simulink model "dcm5"  (R2023a)
settings: Solver=ode45  StartTime=0.0  StopTime=2  RelTol=1e-3  EnableMultiTasking=on
InitFcn:
  | [dcm, cont] = dcm5_init
undefined symbols (not defined in the file or in its folder): cont, dcm
settings Model: Creator=jkempkes  LastModifiedBy=herranz
settings SolverCC: AlgebraicLoopSolver=TrustRegion
settings DataIOCC: LimitDataPoints=on  SaveFormat=Array  SignalLoggingSaveFormat=ModelDataLogs  ReturnWorkspaceOutputs=off  SignalLoggingName=sigsOut
settings OptimizationCC: BooleanDataType=off  LifeSpan=inf
settings DebuggingCC: SaveWithParameterizedLinksMsg=none  UnderspecifiedInitializationDetection=Classic  MergeDetectMultiDrivingBlocksExec=none  SignalResolutionControl=TryResolveAllWithWarning  MultiTaskDSMMsg=warning  MultiTaskCondExecSysMsg=none  UnconnectedInputMsg=warning  UnconnectedOutputMsg=warning  UnconnectedLineMsg=warning  SFUnexpectedBacktrackingDiag=warning  SFNoUnconditionalDefaultTransitionDiag=warning  SFExecutionAtInitializationDiag=none  ArithmeticOperatorsInVariantConditions=warning
settings HardwareCC: ProdBitPerPointer=32  ProdBitPerSizeT=32  ProdBitPerPtrDiffT=32  ProdLargestAtomicFloat=None  ProdIntDivRoundTo=Undefined  ProdEndianess=Unspecified  ProdWordSize=32  ProdHWDeviceType=32-bit Generic  TargetUnknown=on
settings ModelReferenceCC: PropagateSignalLabelsOutOfModel=off
settings SFSimCC: SimUseLocalCustomCode=off  CustomCodeUndefinedFunction=UseInterfaceOnly
settings RTWCC: RTWUseLocalCustomCode=off
settings CodeAppCC: StateflowObjectComments=on
settings GRTTargetCC: TargetLangStandard=C89/C90 (ANSI)  CombineOutputUpdateFcns=off  GRTInterface=on
settings ConfigComp: CovMetricSettings=dw  CovSaveCumulativeToWorkspaceVar=on  CovSaveSingleToWorkspaceVar=on  CovExternalEMLEnable=off

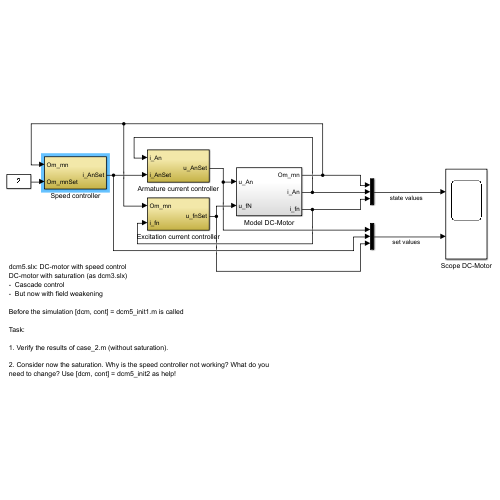
[thumbnail: Simulink's stored preview of the top-level diagram]
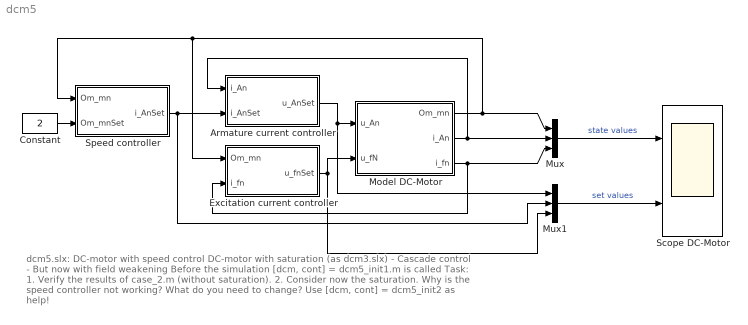
== system dcm5 ==
  note: dcm5.slx: DC-motor with speed control
      | DC-motor with saturation (as dcm3.slx)
      | -  Cascade control
      | -  But now with field weakening
      |
      | Before the simulation [dcm, cont] = dcm5_init1.m is called
      |
      | Task:
      |
      | 1. Verify the results of case_2.m (without saturation).
      |
      | 2. Consider now the saturation. Why is the speed controller not working? What do you need to change? Use [dcm, cont] = dcm5_init2 as help!
  Armature current controller : Subsystem
  Constant : Constant  Value=2
  Excitation current controller : Subsystem
  Model DC-Motor : Subsystem
  Mux : Mux  Inputs=3
  Mux1 : Mux  Inputs=3
  Scope DC-Motor : Scope  NumInputPorts=2
  Speed controller : Subsystem
  wires:
  Mux/1 -> Scope DC-Motor/1  "state values"
  Model DC-Motor/1(Om_mn) -> Mux/1, Speed controller/1(Om_mn), Excitation current controller/1(Om_mn)
  Model DC-Motor/2(i_An) -> Mux/2, Armature current controller/1(i_An)
  Model DC-Motor/3(i_fn) -> Mux/3, Excitation current controller/2(i_fn)
  Speed controller/1(i_AnSet) -> Armature current controller/2(i_AnSet), Mux1/2
  Armature current controller/1(u_AnSet) -> Model DC-Motor/1(u_An), Mux1/1
  Constant/1 -> Speed controller/2(Om_mnSet)
  Excitation current controller/1(u_fnSet) -> Model DC-Motor/2(u_fN), Mux1/3
  Mux1/1 -> Scope DC-Motor/2  "set values"

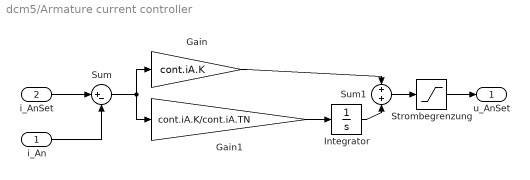
== system dcm5/Armature current controller ==
  i_An : Inport
  i_AnSet : Inport  Port=2
  Gain : Gain  Gain=cont.iA.K  SaturateOnIntegerOverflow=on  OutDataTypeStr=Inherit: Same as input  ParamDataTypeStr=Inherit: Same as input
  Gain1 : Gain  Gain=cont.iA.K/cont.iA.TN  SaturateOnIntegerOverflow=on  OutDataTypeStr=Inherit: Same as input  ParamDataTypeStr=Inherit: Same as input
  Integrator : Integrator  LimitOutput=on  UpperSaturationLimit=cont.u_Anmax  LowerSaturationLimit=-cont.u_Anmax
  Strombegrenzung : Saturate  UpperLimit=cont.u_Anmax  LowerLimit=-cont.u_Anmax
  Sum : Sum  Inputs=|+-  InputSameDT=on  SaturateOnIntegerOverflow=on  OutDataTypeStr=Inherit: Same as first input
  Sum1 : Sum  InputSameDT=on  SaturateOnIntegerOverflow=on  OutDataTypeStr=Inherit: Same as first input
  u_AnSet : Outport  InitialOutput=0
  wires:
  Strombegrenzung/1 -> u_AnSet/1
  i_An/1 -> Sum/2
  Sum/1 -> Gain1/1, Gain/1
  i_AnSet/1 -> Sum/1
  Sum1/1 -> Strombegrenzung/1
  Gain/1 -> Sum1/1
  Integrator/1 -> Sum1/2
  Gain1/1 -> Integrator/1

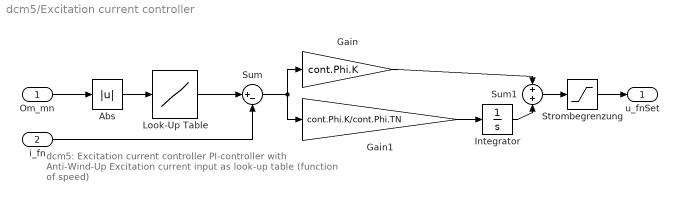
== system dcm5/Excitation current controller ==
  note: dcm5: Excitation current controller
      | PI-controller with Anti-Wind-Up
      | Excitation current input as look-up table (function of speed)
  Om_mn : Inport
  i_fn : Inport  Port=2
  Abs : Abs
  Gain : Gain  Gain=cont.Phi.K  SaturateOnIntegerOverflow=on  OutDataTypeStr=Inherit: Same as input  ParamDataTypeStr=Inherit: Same as input
  Gain1 : Gain  Gain=cont.Phi.K/cont.Phi.TN  SaturateOnIntegerOverflow=on  OutDataTypeStr=Inherit: Same as input  ParamDataTypeStr=Inherit: Same as input
  Integrator : Integrator  InitialCondition=dcm.Pfi_f0  LimitOutput=on  UpperSaturationLimit=cont.u_fnmax  LowerSaturationLimit=0.3*cont.u_fnmax
  Look-Up Table : Lookup  InputValues=cont.LookUpTable.Om  Table=cont.LookUpTable.i_f
  Strombegrenzung : Saturate  UpperLimit=cont.u_fnmax  LowerLimit=0.3*cont.u_fnmax
  Sum : Sum  Inputs=|+-  InputSameDT=on  SaturateOnIntegerOverflow=on  OutDataTypeStr=Inherit: Same as first input
  Sum1 : Sum  InputSameDT=on  SaturateOnIntegerOverflow=on  OutDataTypeStr=Inherit: Same as first input
  u_fnSet : Outport  InitialOutput=0
  wires:
  Strombegrenzung/1 -> u_fnSet/1
  i_fn/1 -> Sum/2
  Sum/1 -> Gain1/1, Gain/1
  Sum1/1 -> Strombegrenzung/1
  Gain/1 -> Sum1/1
  Integrator/1 -> Sum1/2
  Gain1/1 -> Integrator/1
  Look-Up Table/1 -> Sum/1
  Abs/1 -> Look-Up Table/1
  Om_mn/1 -> Abs/1

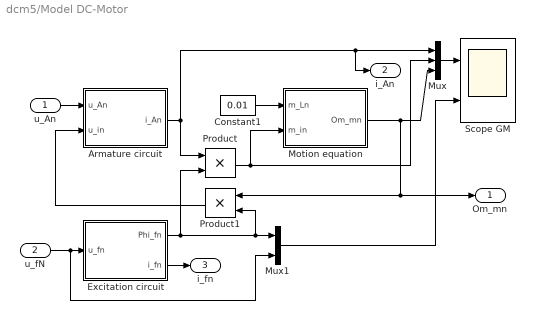
== system dcm5/Model DC-Motor ==
  u_An : Inport
  u_fN : Inport  Port=2
  Armature circuit : Subsystem
  Constant1 : Constant  Value=0.01
  Excitation circuit : Subsystem
  Motion equation : Subsystem
  Mux : Mux  Inputs=3
  Mux1 : Mux  Inputs=2
  Product : Product  InputSameDT=on  SaturateOnIntegerOverflow=on  OutDataTypeStr=Inherit: Same as first input
  Product1 : Product  InputSameDT=on  SaturateOnIntegerOverflow=on  OutDataTypeStr=Inherit: Same as first input
  Scope GM : Scope  NumInputPorts=2
  Om_mn : Outport
  i_An : Outport  Port=2
  i_fn : Outport  Port=3
  wires:
  Armature circuit/1(i_An) -> Product/1, Mux/1, i_An/1
  Excitation circuit/1(Phi_fn) -> Product/2, Product1/2, Mux1/1
  Product/1 -> Motion equation/2(m_in), Mux/2
  Motion equation/1(Om_mn) -> Mux/3, Product1/1, Om_mn/1
  Product1/1 -> Armature circuit/2(u_in)
  Constant1/1 -> Motion equation/1(m_Ln)
  u_fN/1 -> Mux1/2, Excitation circuit/1(u_fn)
  Mux/1 -> Scope GM/1
  Mux1/1 -> Scope GM/2
  u_An/1 -> Armature circuit/1(u_An)
  Excitation circuit/2(i_fn) -> i_fn/1

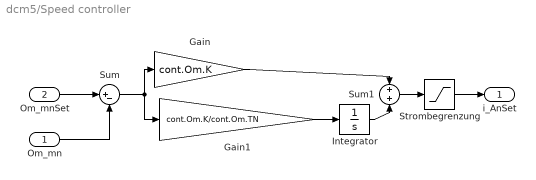
== system dcm5/Speed controller ==
  Om_mn : Inport
  Om_mnSet : Inport  Port=2
  Gain : Gain  Gain=cont.Om.K  SaturateOnIntegerOverflow=on  OutDataTypeStr=Inherit: Same as input  ParamDataTypeStr=Inherit: Same as input
  Gain1 : Gain  Gain=cont.Om.K/cont.Om.TN  SaturateOnIntegerOverflow=on  OutDataTypeStr=Inherit: Same as input  ParamDataTypeStr=Inherit: Same as input
  Integrator : Integrator  LimitOutput=on  UpperSaturationLimit=cont.i_Anmax  LowerSaturationLimit=-cont.i_Anmax
  Strombegrenzung : Saturate  UpperLimit=cont.i_Anmax  LowerLimit=-cont.i_Anmax
  Sum : Sum  Inputs=|+-  InputSameDT=on  SaturateOnIntegerOverflow=on  OutDataTypeStr=Inherit: Same as first input
  Sum1 : Sum  InputSameDT=on  SaturateOnIntegerOverflow=on  OutDataTypeStr=Inherit: Same as first input
  i_AnSet : Outport  InitialOutput=0
  wires:
  Gain1/1 -> Integrator/1
  Integrator/1 -> Sum1/2
  Gain/1 -> Sum1/1
  Sum1/1 -> Strombegrenzung/1
  Om_mnSet/1 -> Sum/1
  Sum/1 -> Gain/1, Gain1/1
  Om_mn/1 -> Sum/2
  Strombegrenzung/1 -> i_AnSet/1

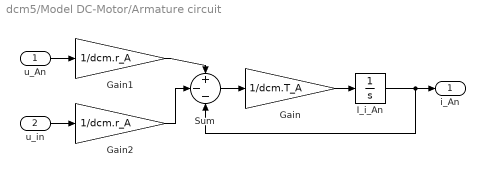
== system dcm5/Model DC-Motor/Armature circuit ==
  u_An : Inport
  u_in : Inport  Port=2
  Gain : Gain  Gain=1/dcm.T_A  SaturateOnIntegerOverflow=on  OutDataTypeStr=Inherit: Same as input  ParamDataTypeStr=Inherit: Same as input
  Gain1 : Gain  Gain=1/dcm.r_A  SaturateOnIntegerOverflow=on  OutDataTypeStr=Inherit: Same as input  ParamDataTypeStr=Inherit: Same as input
  Gain2 : Gain  Gain=1/dcm.r_A  SaturateOnIntegerOverflow=on  OutDataTypeStr=Inherit: Same as input  ParamDataTypeStr=Inherit: Same as input
  I_i_An : Integrator
  Sum : Sum  Inputs=+--  InputSameDT=on  SaturateOnIntegerOverflow=on  OutDataTypeStr=Inherit: Same as first input
  i_An : Outport
  wires:
  Gain/1 -> I_i_An/1
  Sum/1 -> Gain/1
  Gain1/1 -> Sum/1
  Gain2/1 -> Sum/2
  I_i_An/1 -> Sum/3, i_An/1
  u_An/1 -> Gain1/1
  u_in/1 -> Gain2/1

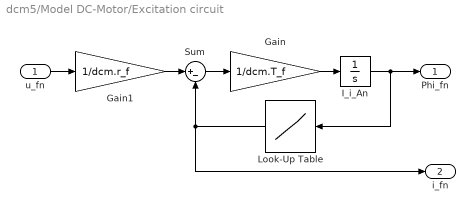
== system dcm5/Model DC-Motor/Excitation circuit ==
  u_fn : Inport
  Gain : Gain  Gain=1/dcm.T_f  SaturateOnIntegerOverflow=on  OutDataTypeStr=Inherit: Same as input  ParamDataTypeStr=Inherit: Same as input
  Gain1 : Gain  Gain=1/dcm.r_f  SaturateOnIntegerOverflow=on  OutDataTypeStr=Inherit: Same as input  ParamDataTypeStr=Inherit: Same as input
  I_i_An : Integrator  InitialCondition=dcm.Pfi_f0
  Look-Up Table : Lookup  InputValues=dcm.Phi_f  Table=dcm.i_f
  Sum : Sum  Inputs=|+-  InputSameDT=on  SaturateOnIntegerOverflow=on  OutDataTypeStr=Inherit: Same as first input
  Phi_fn : Outport
  i_fn : Outport  Port=2
  wires:
  u_fn/1 -> Gain1/1
  I_i_An/1 -> Phi_fn/1, Look-Up Table/1
  Gain1/1 -> Sum/1
  Gain/1 -> I_i_An/1
  Sum/1 -> Gain/1
  Look-Up Table/1 -> Sum/2, i_fn/1

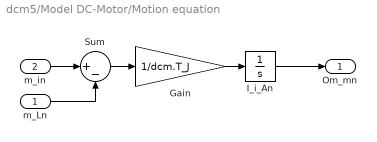
== system dcm5/Model DC-Motor/Motion equation ==
  m_Ln : Inport
  m_in : Inport  Port=2
  Gain : Gain  Gain=1/dcm.T_J  SaturateOnIntegerOverflow=on  OutDataTypeStr=Inherit: Same as input  ParamDataTypeStr=Inherit: Same as input
  I_i_An : Integrator  InitialCondition=dcm.Om_m0
  Sum : Sum  Inputs=|+-  InputSameDT=on  SaturateOnIntegerOverflow=on  OutDataTypeStr=Inherit: Same as first input
  Om_mn : Outport
  wires:
  m_Ln/1 -> Sum/2
  m_in/1 -> Sum/1
  I_i_An/1 -> Om_mn/1
  Sum/1 -> Gain/1
  Gain/1 -> I_i_An/1
